simulink model "TransitionParam"  (R2021b)
settings: Solver=VariableStepAuto  StartTime=0.0  StopTime=10.0  RelTol=1e-3
settings Model: DataDictionary=GuidanceDD.sldd  Creator=lenovo  LastModifiedBy=Paul

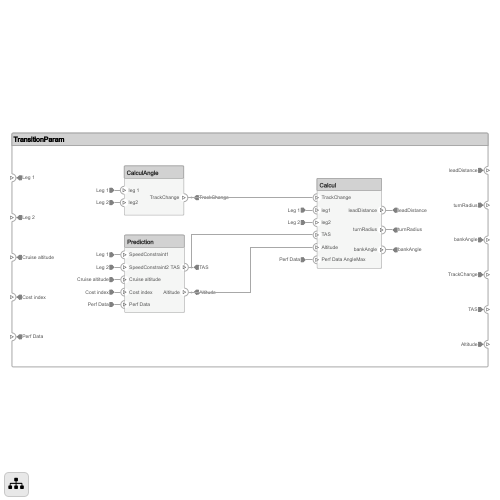
[thumbnail: Simulink's stored preview of the top-level diagram]
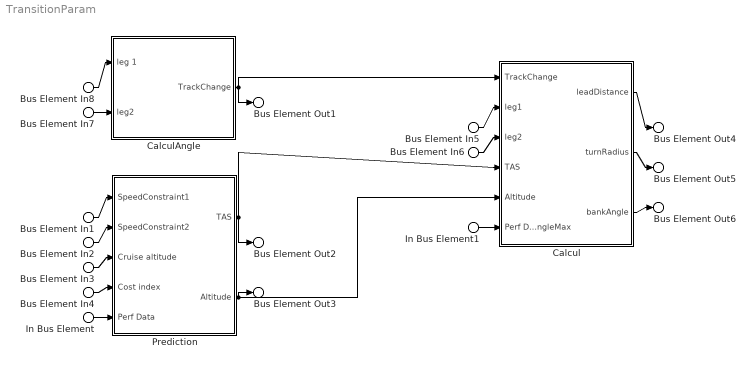
== system TransitionParam ==
  Bus Element In1 : Inport  RequirementInfo={} %GIDa_7e47cab0_69a0_4b41_8527_288de4a17c80  PortName=Leg 1
  Bus Element In5 : Inport  RequirementInfo={} %GIDa_926c13ab_292f_4059_956c_12e77589e20c  PortName=Leg 1
  Bus Element In8 : Inport  RequirementInfo={} %GIDa_c51667d5_aae8_48d8_a40f_bf31e3b72a22  PortName=Leg 1
  Bus Element In2 : Inport  RequirementInfo={} %GIDa_e71f6c8d_6349_40fd_9c80_6af729591ace  Port=2  PortName=Leg 2
  Bus Element In6 : Inport  RequirementInfo={} %GIDa_44df3bda_52e2_4c72_8fb1_862028e7b325  Port=2  PortName=Leg 2
  Bus Element In7 : Inport  RequirementInfo={} %GIDa_3ad87432_05fd_4ba8_81b4_979291bd2c6d  Port=2  PortName=Leg 2
  Bus Element In3 : Inport  RequirementInfo={} %GIDa_26c5fbfc_efe7_49f7_a572_35e02195aa60  Port=3  PortName=Cruise altitude
  Bus Element In4 : Inport  RequirementInfo={} %GIDa_c7dd64a4_29f3_4dd6_9876_9123f4993590  Port=4  PortName=Cost index
  In Bus Element : Inport  Port=5  PortName=Perf Data
  In Bus Element1 : Inport  Port=5  PortName=Perf Data
  Calcul : Subsystem  RequirementInfo={} %GIDa_e63fb47b_7466_419f_802c_7578e2e7b7d8
      settings: PortSchema="{\"entries\":[{\"content\":{\"headerSize\":26,\"margin\":15,\"minimumSpacing\":25,\"sides\":[{\"content\":{\"connectorIds\":[\"In2\",\"In3\",\"In4\",\"In1\",\"In5\",\"In6\"]},\"type\":\"ConnectorPlacement.EquallySpacedRectSide\",\"uuid\":\"1fe9f491-8940-4068-a798-04a3b940f4fc\"},{\"content\":{\"connectorIds\":[\"Out1\",\"Out2\",\"Out3\"],\"side\":\"RIGHT\"},\"type\":\"ConnectorPlacement.EquallySpacedRectSide\",\"uuid\":\"599ca7dc-45bb-4841-abdf-2264bce8800e\"},{\"content\":{\"connectorIds\":[],\"side\":\"TOP\"},\"type\":\"ConnectorPlacement.EquallySpacedRectSide\",\"uuid\":\"c53441a1-491c-45f7-94f0-5f364038b604\"}]},\"type\":\"ConnectorPlacement.EquallySpacedConnector\",\"uuid\":\"79cb965a-071d-4caa-a027-7b08a0e7657c\"}],\"packageUris\":[\"http://schema.mathworks.com/mf0/Connector/R2020b\"],\"version\":\"1.0\"}"
  CalculAngle : Subsystem  RequirementInfo={} %GIDa_42e67d5b_b337_4844_8632_52dfdd222e57
      settings: PortSchema="{\"entries\":[{\"content\":{\"headerSize\":26,\"margin\":15,\"minimumSpacing\":25,\"sides\":[{\"content\":{\"connectorIds\":[\"In1\",\"In2\"]},\"type\":\"ConnectorPlacement.EquallySpacedRectSide\",\"uuid\":\"1fe9f491-8940-4068-a798-04a3b940f4fc\"},{\"content\":{\"connectorIds\":[\"Out1\"],\"side\":\"RIGHT\"},\"type\":\"ConnectorPlacement.EquallySpacedRectSide\",\"uuid\":\"599ca7dc-45bb-4841-abdf-2264bce8800e\"},{\"content\":{\"connectorIds\":[],\"side\":\"TOP\"},\"type\":\"ConnectorPlacement.EquallySpacedRectSide\",\"uuid\":\"c53441a1-491c-45f7-94f0-5f364038b604\"}]},\"type\":\"ConnectorPlacement.EquallySpacedConnector\",\"uuid\":\"79cb965a-071d-4caa-a027-7b08a0e7657c\"}],\"packageUris\":[\"http://schema.mathworks.com/mf0/Connector/R2020b\"],\"version\":\"1.0\"}"
  Prediction : Subsystem  RequirementInfo={} %GIDa_bfee97b2_c03d_4999_96e8_b69180879f4a
      settings: PortSchema="{\"entries\":[{\"content\":{\"headerSize\":26,\"margin\":15,\"minimumSpacing\":25,\"sides\":[{\"content\":{\"connectorIds\":[\"In1\",\"In2\",\"In3\",\"In4\",\"In5\"]},\"type\":\"ConnectorPlacement.EquallySpacedRectSide\",\"uuid\":\"6cd795b8-c074-4b6c-9624-28530f1ec42c\"},{\"content\":{\"connectorIds\":[\"Out1\",\"Out2\"],\"side\":\"RIGHT\"},\"type\":\"ConnectorPlacement.EquallySpacedRectSide\",\"uuid\":\"705c6af3-08cf-4cab-b41a-726488ec4b4a\"},{\"content\":{\"connectorIds\":[],\"side\":\"TOP\"},\"type\":\"ConnectorPlacement.EquallySpacedRectSide\",\"uuid\":\"5691381f-82f1-4417-8811-ac3c480a5de6\"}]},\"type\":\"ConnectorPlacement.EquallySpacedConnector\",\"uuid\":\"1acf3cee-d226-4abb-ac39-1c752c6f4ef7\"}],\"packageUris\":[\"http://schema.mathworks.com/mf0/Connector/R2020b\"],\"version\":\"1.0\"}"
  Bus Element Out4 : Outport  RequirementInfo={} %GIDa_21bc16ce_2261_41b6_be60_cad84dff5095  PortName=leadDistance
  Bus Element Out5 : Outport  RequirementInfo={} %GIDa_764184ef_ba28_4725_9e1a_3116edc4ded6  Port=2  PortName=turnRadius
  Bus Element Out6 : Outport  RequirementInfo={} %GIDa_ad323867_5aef_4ed3_912a_86a7715b4ece  Port=3  PortName=bankAngle
  Bus Element Out1 : Outport  RequirementInfo={} %GIDa_81d0ff53_c706_4f68_a58d_135195926998  Port=4  PortName=TrackChange
  Bus Element Out2 : Outport  RequirementInfo={} %GIDa_2a4c0edc_bad2_4298_871e_e9a084d12293  Port=5  PortName=TAS
  Bus Element Out3 : Outport  RequirementInfo={} %GIDa_130d8a00_ae83_4ea9_ad6f_148b951198f4  Port=6  PortName=Altitude
  wires:
  CalculAngle/1(TrackChange) -> Calcul/2(TrackChange), Bus Element Out1/1
  Bus Element In3/1 -> Prediction/3(Cruise altitude)
  Bus Element In4/1 -> Prediction/4(Cost index)
  Bus Element In1/1 -> Prediction/1(SpeedConstraint1)
  Bus Element In2/1 -> Prediction/2(SpeedConstraint2)
  Prediction/1(TAS) -> Calcul/1(TAS), Bus Element Out2/1
  Prediction/2(Altitude) -> Calcul/5(Altitude), Bus Element Out3/1
  Calcul/1(leadDistance) -> Bus Element Out4/1
  Calcul/2(turnRadius) -> Bus Element Out5/1
  Calcul/3(bankAngle) -> Bus Element Out6/1
  Bus Element In5/1 -> Calcul/3(leg1)
  Bus Element In6/1 -> Calcul/4(leg2)
  Bus Element In7/1 -> CalculAngle/2(leg2)
  Bus Element In8/1 -> CalculAngle/1(leg 1)
  In Bus Element/1 -> Prediction/5(Perf Data)
  In Bus Element1/1 -> Calcul/6(Perf Data AngleMax)

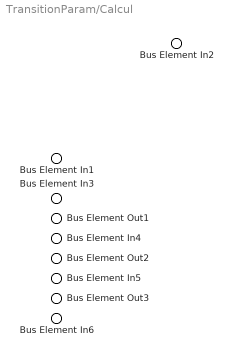
== system TransitionParam/Calcul ==
  Bus Element In2 : Inport  RequirementInfo={} %GIDa_6ac94ae8_d44e_49c8_92b8_134695fa8b1d  PortName=TAS
  Bus Element In1 : Inport  RequirementInfo={} %GIDa_93fac0ec_a76a_4d1e_bfb2_73d3b4b4d998  Port=2  PortName=TrackChange
  Bus Element In3 : Inport  RequirementInfo={} %GIDa_2be217fc_1106_47fa_88ec_8d95c597d98f  Port=3  PortName=leg1
  Bus Element In4 : Inport  RequirementInfo={} %GIDa_54775a5f_4274_4c5b_8f20_49e03b85e931  Port=4  PortName=leg2
  Bus Element In5 : Inport  RequirementInfo={} %GIDa_6e2c9de9_6abe_45ad_abfc_d09754817925  Port=5  PortName=Altitude
  Bus Element In6 : Inport  Port=6  PortName=Perf Data AngleMax
  Bus Element Out1 : Outport  RequirementInfo={} %GIDa_4edb4009_c062_4ca5_b8d2_8a38d56858aa  PortName=leadDistance
  Bus Element Out2 : Outport  RequirementInfo={} %GIDa_51636c58_f267_48e6_acd9_c82a005e020e  Port=2  PortName=turnRadius
  Bus Element Out3 : Outport  RequirementInfo={} %GIDa_38b5f455_20d4_488e_af80_5f9344afc940  Port=3  PortName=bankAngle

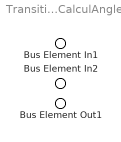
== system TransitionParam/CalculAngle ==
  Bus Element In1 : Inport  RequirementInfo={} %GIDa_b985d850_646e_41b5_8941_cf259979ddf1  PortName=leg 1
  Bus Element In2 : Inport  RequirementInfo={} %GIDa_d93819e3_2170_4e6d_b5e4_4e7efcfdf2be  Port=2  PortName=leg2
  Bus Element Out1 : Outport  RequirementInfo={} %GIDa_62121e54_66ae_418b_9497_4ddac0debed6  PortName=TrackChange

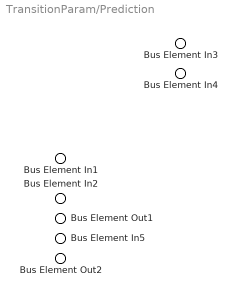
== system TransitionParam/Prediction ==
  Bus Element In3 : Inport  RequirementInfo={} %GIDa_825df91d_8fe3_4996_b693_5d74cbe14620  PortName=SpeedConstraint1
  Bus Element In4 : Inport  RequirementInfo={} %GIDa_d5330151_3445_4611_9bb2_f8cbaf71c905  Port=2  PortName=SpeedConstraint2
  Bus Element In1 : Inport  RequirementInfo={} %GIDa_0f37a200_f8d4_4b30_8555_d766b3477f48  Port=3  PortName=Cruise altitude
  Bus Element In2 : Inport  RequirementInfo={} %GIDa_96d27252_759f_4780_9388_d415d38c26e4  Port=4  PortName=Cost index
  Bus Element In5 : Inport  Port=5  PortName=Perf Data
  Bus Element Out1 : Outport  RequirementInfo={} %GIDa_89e912dd_3116_407e_8344_d46ea1f84145  PortName=TAS
  Bus Element Out2 : Outport  RequirementInfo={} %GIDa_6c23f067_53e1_4764_9fd4_ac04394c972f  Port=2  PortName=Altitude
